simulink model "CellVoltageDiagnostics_MIL_Test"  (R2022b)
settings: Solver=FixedStepAuto  StartTime=0.0  StopTime=inf  FixedStep=TsBatt  RelTol=1e-3  EnableMultiTasking=on
PreLoadFcn:
  | ts = 0.1;
libraries: fl_lib x10, nesl_utility x10, BatteryPack_lib x1
settings Model: DataDictionary=Shared_DD_TMS570.sldd  sg_rtwmakecfg_data=_PIL_HWD__Pilpxi__sglibc_  PacingRate=10  Creator=cpatel  LastModifiedBy=mathieu.lu-dac
settings SolverCC: ConcurrentTasks=on  AlgebraicLoopSolver=TrustRegion  PositivePriorityOrder=on  AutoInsertRateTranBlk=on  InsertRTBMode=Never (minimum delay)
settings DataIOCC: SaveFormat=StructureWithTime
settings OptimizationCC: BlockReduction=off  UseFloatMulNetSlope=on  OptimizeBlockIOStorage=off  BufferReuse=off  GlobalBufferReuse=off  ExpressionFolding=off  LocalBlockOutputs=off  OptimizeDataStoreBuffers=off  BusAssignmentInplaceUpdate=off
settings DebuggingCC: TasksWithSamePriorityMsg=none  UnconnectedInputMsg=warning  UnconnectedOutputMsg=warning  UnconnectedLineMsg=warning  SFMachineParentedDataDiag=warning  ArithmeticOperatorsInVariantConditions=warning
settings HardwareCC: ProdBitPerLong=64  ProdLongLongMode=on  ProdHWDeviceType=Intel->x86-64 (Linux 64)
settings ModelReferenceCC: EnableRefExpFcnMdlSchedulingChecks=on  ModelReferenceNumInstancesAllowed=Single
settings SFSimCC: MATLABDynamicMemAlloc=off  CustomCodeUndefinedFunction=UseInterfaceOnly
settings RTWCC: Description=Simulink Real-Time  SystemTargetFile=slrealtime.tlc  TemplateMakefile=slrealtime_default_tmf  Toolchain=Simulink Real-Time Toolchain  BuildConfiguration=Faster Runs  CodeExecutionProfiling=on  TargetLang=C++  DLArmComputeVersion=19.05
settings CodeAppCC: MaxIdLength=51
settings SimulinkRealTimeTargetCC: UseGCCFastMath=on

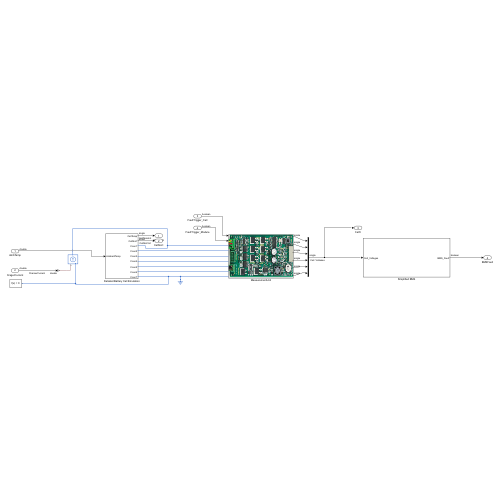
[thumbnail: Simulink's stored preview of the top-level diagram]
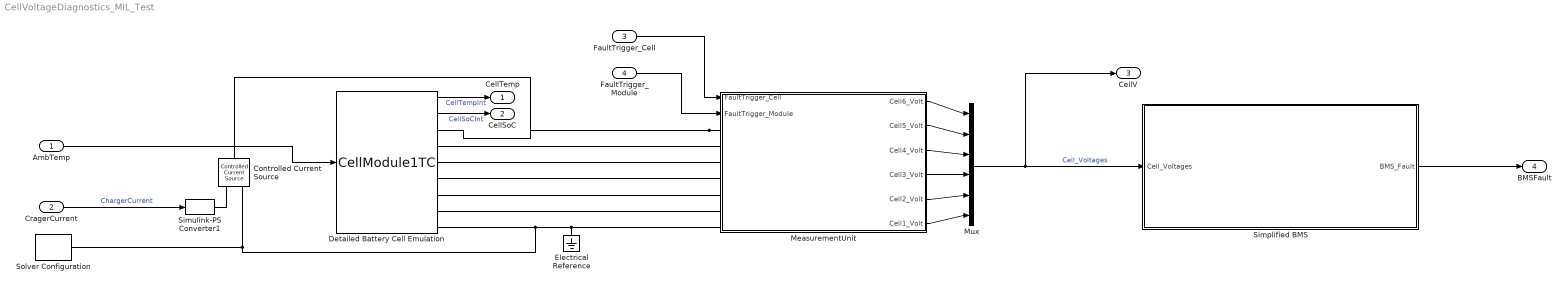
== system CellVoltageDiagnostics_MIL_Test ==
  AmbTemp : Inport  Unit=K
  CragerCurrent : Inport  Port=2
  FaultTrigger_Cell : Inport  Port=3  OutDataTypeStr=boolean
  FaultTrigger_Module : Inport  Port=4  OutDataTypeStr=boolean
  Controlled Current Source : fl_lib/Electrical/Electrical Sources/Controlled Current Source
      settings: LogSimulationData=on
  Detailed Battery Cell Emulation : BatteryPack_lib/CellModule1TC  SystemSampleTime=-1  VariantActivationTime=update diagram  Latency=0  AutoFrameSizeCalculation=off
  Electrical Reference : fl_lib/Electrical/Electrical Elements/Electrical Reference
  MeasurementUnit : Subsystem
      mask Display: image('TCU.png');
  Mux : Mux  Inputs=6
  Simplified BMS : Subsystem
  Simulink-PS Converter1 : nesl_utility/Simulink-PS Converter  PhysicalDomain=network_engine_domain  SubClassName=ps_input  LeftPortType=input  RightPortType=output  PseudoPeriodic=off  Frequencies=[]  NoiseDistribution=none  NoiseParameters=[]  Unit=1  AffineConversion=off  FilteringAndDerivatives=zero  SimscapeFilterOrder=1  InputFilterTimeConstant=0.001  UdotUserProvided=1
  Solver Configuration : nesl_utility/Solver Configuration  PhysicalDomain=network_engine_domain  SubClassName=solver  LeftPortType=input  RightPortType=generic  Tones=[]  Harmonics=[]  SimulateNoise=off  Profile=off  UseLocalSampling=off  EnableSwitchedLinearOptims=on  FrequencyDomain=off  UseCCode=off  RelTol=0.001  AbsTol=1e-06  MinStep=1e-09  ToWorkspace=off  RevertToSquareIcSolve=off  NumHomotopyIterations=100  PhasorMode=off  PhasorModeNumHarmonics=1  ConsistencySolver=NEWTON_FTOL  IndexReductionMethod=DerivativeReplacement  DoDC=off  ResidualTolerance=1e-09  ConsistencyTolSource=GLOBAL  ConsistencyAbsTol=0.001  ConsistencyRelTol=0.001  ConsistencyTolFactor=0.001  UseLocalSolver=on  LocalSolverChoice=NE_BACKWARD_EULER_ADVANCER  ResolveIndetEquations=on  FunctionEvalNumThread=1  LocalSolverSampleTime=TsBatt  DoFixedCost=on  MaxNonlinIter=3  MaxModeIter=2  ComputeImpulses=off  ImpulseIterations=2  LinearAlgebra=auto  LinearAlgebraNumThread=0  EquationFormulation=NE_TIME_EF  DelaysMemoryBudget=1024  AutomaticFiltering=on  FilteringTimeConstant=0.001  PartitionStorageMethod=AS_NEEDED  PartitionMemoryBudget=1024  PartitionMethod=ROBUST
  CellTemp : Outport
  CellSoC : Outport  Port=2
  CellV : Outport  Port=3
  BMSFault : Outport  Port=4
  wires:
  Detailed Battery Cell Emulation/1 -> CellTemp/1  "CellTempInt"
  Detailed Battery Cell Emulation/2 -> CellSoC/1  "CellSoCInt"
  MeasurementUnit/6(Cell1_Volt) -> Mux/6
  FaultTrigger_Cell/1 -> MeasurementUnit/1(FaultTrigger_Cell)
  MeasurementUnit/3(Cell4_Volt) -> Mux/3
  MeasurementUnit/1(Cell6_Volt) -> Mux/1
  MeasurementUnit/5(Cell2_Volt) -> Mux/5
  MeasurementUnit/4(Cell3_Volt) -> Mux/4
  MeasurementUnit/2(Cell5_Volt) -> Mux/2
  AmbTemp/1 -> Detailed Battery Cell Emulation/1
  CragerCurrent/1 -> Simulink-PS Converter1/1  "ChargerCurrent"
  Mux/1 -> Simplified BMS/1(Cell_Voltages), CellV/1  "Cell_Voltages"
  Simplified BMS/1(BMS_Fault) -> BMSFault/1
  FaultTrigger_Module/1 -> MeasurementUnit/2(FaultTrigger_Module)
  connections:
  Controlled Current Source/RConn2 -- Solver Configuration/RConn1 -- Detailed Battery Cell Emulation/RConn7 -- MeasurementUnit/LConn7 -- Electrical Reference/LConn1
  MeasurementUnit/LConn1 -- Detailed Battery Cell Emulation/RConn1 -- Controlled Current Source/LConn1
  Detailed Battery Cell Emulation/RConn6 -- MeasurementUnit/LConn6
  Detailed Battery Cell Emulation/RConn5 -- MeasurementUnit/LConn5
  Detailed Battery Cell Emulation/RConn4 -- MeasurementUnit/LConn4
  Simulink-PS Converter1/RConn1 -- Controlled Current Source/RConn1
  Detailed Battery Cell Emulation/RConn3 -- MeasurementUnit/LConn3
  Detailed Battery Cell Emulation/RConn2 -- MeasurementUnit/LConn2

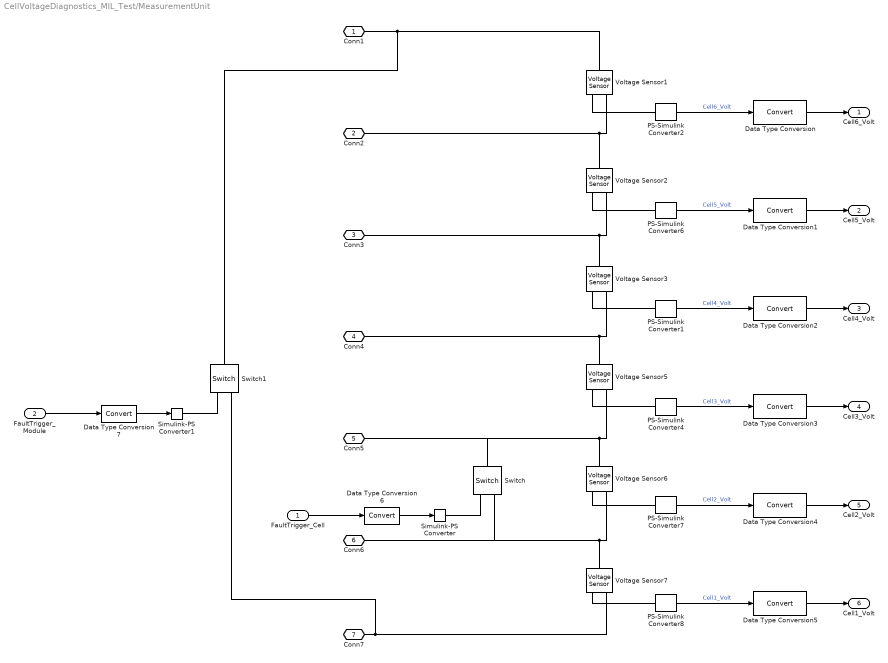
== system CellVoltageDiagnostics_MIL_Test/MeasurementUnit ==
  FaultTrigger_Cell : Inport
  FaultTrigger_Module : Inport  Port=2
  Data Type Conversion{,1..7} (8 alike) : DataTypeConversion  SaturateOnIntegerOverflow=off  RndMeth=Floor
  PS-Simulink Converter{1..2,4,6..8} (6 alike) : nesl_utility/PS-Simulink Converter  PhysicalDomain=network_engine_domain  SubClassName=ps_output  LeftPortType=input  RightPortType=output  PseudoPeriodic=off  Frequencies=[]  VectorFormat=1-D array  Unit=V  AffineConversion=off
  Simulink-PS Converter : nesl_utility/Simulink-PS Converter  PhysicalDomain=network_engine_domain  SubClassName=ps_input  LeftPortType=input  RightPortType=output  PseudoPeriodic=off  Frequencies=[]  NoiseDistribution=none  NoiseParameters=[]  Unit=1  AffineConversion=off  FilteringAndDerivatives=provide  SimscapeFilterOrder=1  InputFilterTimeConstant=0.001  UdotUserProvided=0
  Simulink-PS Converter1 : nesl_utility/Simulink-PS Converter  PhysicalDomain=network_engine_domain  SubClassName=ps_input  LeftPortType=input  RightPortType=output  PseudoPeriodic=off  Frequencies=[]  NoiseDistribution=none  NoiseParameters=[]  Unit=1  AffineConversion=off  FilteringAndDerivatives=provide  SimscapeFilterOrder=1  InputFilterTimeConstant=0.001  UdotUserProvided=0
  Switch : fl_lib/Electrical/Electrical Elements/Switch  R_closed=0.01 Ohm  G_open=1e-8 1/Ohm  Threshold=0.5  i_specify=off  i_priority=None  i=0 A  i_nominal_specify=off  i_nominal_unit=A  i_nominal_value=1  v_specify=off  v_priority=None  v=0 V  v_nominal_specify=off  v_nominal_unit=V  v_nominal_value=1
  Switch1 : fl_lib/Electrical/Electrical Elements/Switch  R_closed=0.01 Ohm  G_open=1e-8 1/Ohm  Threshold=0.5  i_specify=off  i_priority=None  i=0 A  i_nominal_specify=off  i_nominal_unit=A  i_nominal_value=1  v_specify=off  v_priority=None  v=0 V  v_nominal_specify=off  v_nominal_unit=V  v_nominal_value=1
  Voltage Sensor{1..3,5..7} (6 alike) : fl_lib/Electrical/Electrical Sensors/Voltage Sensor
  Conn1 : PMIOPort  Side=Left
  Conn2 : PMIOPort  Port=2  Side=Left
  Conn3 : PMIOPort  Port=3  Side=Left
  Conn4 : PMIOPort  Port=4  Side=Left
  Conn5 : PMIOPort  Port=5  Side=Left
  Conn6 : PMIOPort  Port=6  Side=Left
  Conn7 : PMIOPort  Port=7  Side=Left
  Cell6_Volt : Outport  VectorParamsAs1DForOutWhenUnconnected=off
  Cell5_Volt : Outport  Port=2  VectorParamsAs1DForOutWhenUnconnected=off
  Cell4_Volt : Outport  Port=3  VectorParamsAs1DForOutWhenUnconnected=off
  Cell3_Volt : Outport  Port=4  VectorParamsAs1DForOutWhenUnconnected=off
  Cell2_Volt : Outport  Port=5  VectorParamsAs1DForOutWhenUnconnected=off
  Cell1_Volt : Outport  Port=6  VectorParamsAs1DForOutWhenUnconnected=off
  wires:
  PS-Simulink Converter1/1 -> Data Type Conversion2/1  "Cell4_Volt"
  PS-Simulink Converter7/1 -> Data Type Conversion4/1  "Cell2_Volt"
  PS-Simulink Converter2/1 -> Data Type Conversion/1  "Cell6_Volt"
  PS-Simulink Converter4/1 -> Data Type Conversion3/1  "Cell3_Volt"
  PS-Simulink Converter8/1 -> Data Type Conversion5/1  "Cell1_Volt"
  PS-Simulink Converter6/1 -> Data Type Conversion1/1  "Cell5_Volt"
  Data Type Conversion/1 -> Cell6_Volt/1
  Data Type Conversion1/1 -> Cell5_Volt/1
  Data Type Conversion2/1 -> Cell4_Volt/1
  Data Type Conversion3/1 -> Cell3_Volt/1
  Data Type Conversion5/1 -> Cell1_Volt/1
  Data Type Conversion4/1 -> Cell2_Volt/1
  FaultTrigger_Cell/1 -> Data Type Conversion6/1
  Data Type Conversion6/1 -> Simulink-PS Converter/1
  Data Type Conversion7/1 -> Simulink-PS Converter1/1
  FaultTrigger_Module/1 -> Data Type Conversion7/1
  connections:
  PS-Simulink Converter2/LConn1 -- Voltage Sensor1/RConn1
  Voltage Sensor2/LConn1 -- Voltage Sensor1/RConn2 -- Conn2/RConn1
  Voltage Sensor6/RConn2 -- Switch/RConn2 -- Conn6/RConn1 -- Voltage Sensor7/LConn1
  Voltage Sensor5/RConn1 -- PS-Simulink Converter4/LConn1
  Voltage Sensor7/RConn1 -- PS-Simulink Converter8/LConn1
  Voltage Sensor5/LConn1 -- Voltage Sensor3/RConn2 -- Conn4/RConn1
  Voltage Sensor6/LConn1 -- Conn5/RConn1 -- Switch/LConn1 -- Voltage Sensor5/RConn2
  Voltage Sensor3/LConn1 -- Voltage Sensor2/RConn2 -- Conn3/RConn1
  Voltage Sensor6/RConn1 -- PS-Simulink Converter7/LConn1
  Voltage Sensor2/RConn1 -- PS-Simulink Converter6/LConn1
  Voltage Sensor3/RConn1 -- PS-Simulink Converter1/LConn1
  Voltage Sensor1/LConn1 -- Switch1/LConn1 -- Conn1/RConn1
  Voltage Sensor7/RConn2 -- Switch1/RConn2 -- Conn7/RConn1
  Switch/RConn1 -- Simulink-PS Converter/RConn1
  Switch1/RConn1 -- Simulink-PS Converter1/RConn1

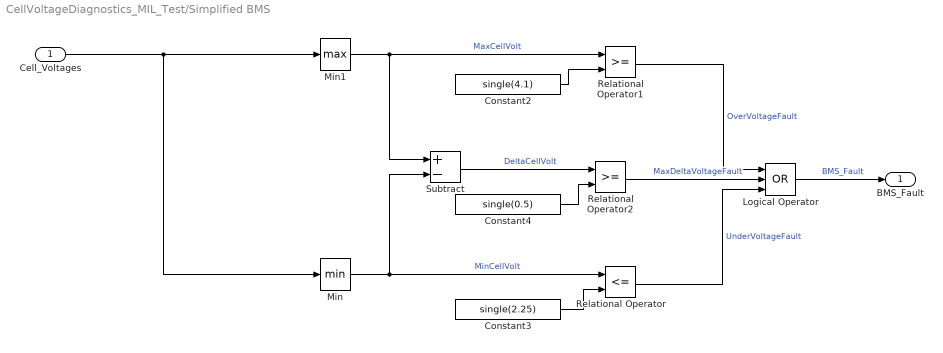
== system CellVoltageDiagnostics_MIL_Test/Simplified BMS ==
  Cell_Voltages : Inport
  Constant2 : Constant  Value=single(4.1)
  Constant3 : Constant  Value=single(2.25)
  Constant4 : Constant  Value=single(0.5)
  Logical Operator : Logic  Operator=OR  Inputs=3  AllPortsSameDT=off  OutDataTypeStr=boolean
  Min : MinMax
  Min1 : MinMax  Function=max
  Relational Operator : RelationalOperator  Operator=<=  OutDataTypeStr=boolean  RndMeth=Simplest  InputSameDT=off
  Relational Operator1 : RelationalOperator  OutDataTypeStr=boolean  RndMeth=Simplest  InputSameDT=off
  Relational Operator2 : RelationalOperator  OutDataTypeStr=boolean  RndMeth=Simplest  InputSameDT=off
  Subtract : Sum  Inputs=+-
  BMS_Fault : Outport
  wires:
  Constant3/1 -> Relational Operator/2
  Logical Operator/1 -> BMS_Fault/1  "BMS_Fault"
  Constant4/1 -> Relational Operator2/2
  Min1/1 -> Subtract/1, Relational Operator1/1  "MaxCellVolt"
  Constant2/1 -> Relational Operator1/2
  Relational Operator/1 -> Logical Operator/3  "UnderVoltageFault"
  Min/1 -> Subtract/2, Relational Operator/1  "MinCellVolt"
  Subtract/1 -> Relational Operator2/1  "DeltaCellVolt"
  Relational Operator1/1 -> Logical Operator/1  "OverVoltageFault"
  Relational Operator2/1 -> Logical Operator/2  "MaxDeltaVoltageFault"
  Cell_Voltages/1 -> Min/1, Min1/1
